simulink model "untitled"  (R2023a)
settings: Solver=VariableStepAuto  StartTime=0.0  StopTime=10.0  RelTol=1e-3
undefined symbols (not defined in the file or in its folder): fft1, ifft1, mmc2
libraries: dspvision x2
settings Model: Creator=Rifat  LastModifiedBy=mrand
settings SolverCC: AlgebraicLoopSolver=TrustRegion
settings DebuggingCC: UnconnectedInputMsg=warning  UnconnectedOutputMsg=warning  UnconnectedLineMsg=warning
settings ModelReferenceCC: EnableRefExpFcnMdlSchedulingChecks=on

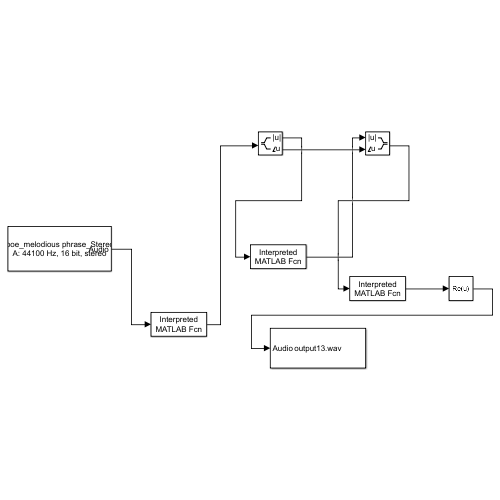
[thumbnail: Simulink's stored preview of the top-level diagram]
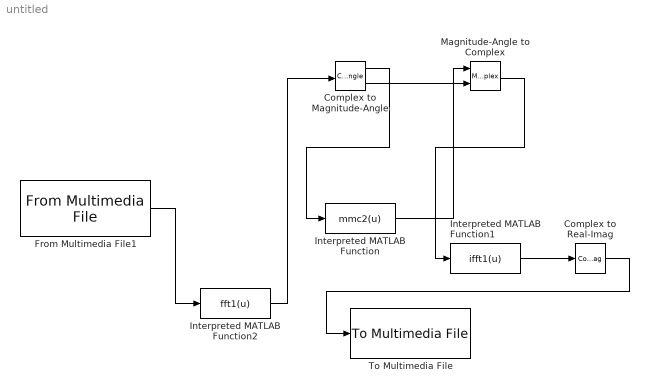
== system untitled ==
  Complex to Magnitude-Angle : ComplexToMagnitudeAngle
  Complex to Real-Imag : ComplexToRealImag  Output=Real
  From Multimedia File1 : dspvision/From Multimedia File  inputFilename=G:\Мой диск\УЧЕБА\Мага\2 курс\2.2_АСД\!!!MATLAB\13 Oboe_melodious phrase_Stereo.wav  readRange=[1 Inf]  loop=on  numPlays=inf  outputStreams=Audio only  videoDataType=single  audioDataType=double  inheritSampleTime=on  userDefinedSampleTime=1/30  noAudioOutput=off  isIntensityVideo=off  fourcc=RGB  colorVideoFormat=Separate color signals  outputEOF=off  dataOrg=Column-major  audioFrameSize=1024  computeAudioFrameSize=off  outSamplingMode=Sample based
  Interpreted MATLAB Function : MATLABFcn  MATLABFcn=mmc2(u)  Output1D=off
  Interpreted MATLAB Function1 : MATLABFcn  MATLABFcn=ifft1(u)  Output1D=off
  Interpreted MATLAB Function2 : MATLABFcn  MATLABFcn=fft1(u)  Output1D=off
  Magnitude-Angle to Complex : MagnitudeAngleToComplex
  To Multimedia File : dspvision/To Multimedia File  outputFilename=output13.wav  streamSelection=Audio only  videoCompressor=None (uncompressed)  audioCompressor=None (uncompressed)  imagePorts=Separate color signals  fileType=WAV  audioDatatype=Determine from input data type  fourcc=RGB  videoQuality=75  mj2000CompFactor=10
  wires:
  From Multimedia File1/1 -> Interpreted MATLAB Function2/1
  Interpreted MATLAB Function2/1 -> Complex to Magnitude-Angle/1
  Interpreted MATLAB Function/1 -> Magnitude-Angle to Complex/1
  Magnitude-Angle to Complex/1 -> Interpreted MATLAB Function1/1
  Interpreted MATLAB Function1/1 -> Complex to Real-Imag/1
  Complex to Real-Imag/1 -> To Multimedia File/1
  Complex to Magnitude-Angle/1 -> Interpreted MATLAB Function/1
  Complex to Magnitude-Angle/2 -> Magnitude-Angle to Complex/2
